simulink model "Commande_7_ReglageCascade_Hinf"  (R2015a)
settings: Solver=ode45  StartTime=0.0  StopTime=20  RelTol=1e-3
values from neighbouring files (symbols this model uses):
  K = place(Aze,Bze,P)    [A_2_Changement_de_base_Diphiomorphisme.m]    (also in A_3_LoopShaping.m = 5000)
  Kd = p1^2*J4    (= 0.0333)    [A_1_Data.m]    (also in matlab.mat = 0.009)
  Kp = -2*p1*J4    (= 0.00222)    [A_1_Data.m]    (also in matlab.mat = 0.0006)
  s = tf('s')    [A_3_LoopShaping.m]    (also in A_4_Hinfini.m = zpk('s'))
  X = [0;0;0;0;0;0;0;0]    [A_1_Data.m]
  Y = [0;0;0;0;0;0;0;0]    [A_1_Data.m]
undefined symbols (not defined in the file or in its folder): Z
libraries: sm_lib x332, nesl_utility x15, simulink x1
(part 8 of 10)

== system Commande_7_ReglageCascade_Hinf/RDelta_SM/RD_SM2/BrasParalelle1/BarreParalleles_2_RIGID/Pice4_Tube_1_RIGID ==
  ReferenceFrame : sm_lib/Frames and Transforms/Reference Frame  BlockFunction=simmechanics.library.frames_transforms.reference_frame
  Solid : sm_lib/Body Elements/Solid  InertiaType=Custom  Mass=0.0056953775725032503  MassUnits=kg  CenterOfMass=[-4.1460122344799134e-11 2.6332345173922464e-08 157.00037492761294]  CenterOfMassUnits=mm  MomentsOfInertia=[46.656669534748204 46.656784060773653 0.060513437161415502]  MomentsOfInertiaUnits=kg*mm^2  ProductsOfInertia=[4.4271388779002391e-06 -1.0344554341986986e-06 -6.5578304138838094e-07]  ProductsOfInertiaUnits=kg*mm^2  DensityBased=on  Density=1000  DensityUnits=kg/(m^3)  GraphicType=FromGeometry  MarkerShape=Sphere  MarkerSize=10  MarkerSizeUnits=m  GraphicVisPropType=SimpleVisualProperties  GraphicDiffuseColor=[0.0 0.0 0.0]  GraphicSpecularColor=[0.5 0.5 0.5 1.0]  GraphicAmbientColor=[0.15 0.15 0.15 1.0]  GraphicEmissiveColor=[1.0 0.0 0.0 1.0]  GraphicShininess=75  GraphicOpacity=1  GeometryShape=FromFile  RectangleSize=[1 1]  RectangleSizeUnits=m  BrickDimensions=[1 1 1]  BrickDimensionUnits=m  CylinderRadius=1  CylinderRadiusUnits=m  CylinderLength=1  CylinderLengthUnits=m  SphereRadius=1  SphereRadiusUnits=m  EllipsoidRadii=[1 1 1]  EllipsoidRadiiUnits=m  ExtrusionCrossSection=[1 1; -1 1; -1 -1; 1 -1]  ExtrusionCrossSectionUnits=m  ExtrusionLength=1  ExtrusionLengthUnits=m  PolygonNumSides=3  PolygonOuterRadius=1  PolygonOuterRadiusUnits=m  ExtGeomFileType=STL  ExtGeomFileName=Pièce4_Tube_Défaut_sldprt.STL  ExtGeomFileUnits=mm  RevolutionCrossSection=[1 1; 1 -1; 2 -1; 2 1]  RevolutionCrossSectionUnits=m  RevolutionExtent=Full  RevolutionAngle=180  RevolutionAngleUnits=deg  BlockFunction=simmechanics.library.body_elements.solid
  F : PMIOPort  Port=1  Side=Left
  connections:
  Solid/RConn1 -- ReferenceFrame/RConn1 -- F/RConn1

== system Commande_7_ReglageCascade_Hinf/RDelta_SM/RD_SM2/BrasParalelle2/BarreParalleles_1_RIGID/Pice4_Extremetees_1_RIGID ==
  ReferenceFrame : sm_lib/Frames and Transforms/Reference Frame  BlockFunction=simmechanics.library.frames_transforms.reference_frame
  Solid : sm_lib/Body Elements/Solid  InertiaType=Custom  Mass=0.0043409919402835973  MassUnits=kg  CenterOfMass=[-6.6394731011390018e-06 -1.3723999560385911 4.9969803448403587]  CenterOfMassUnits=mm  MomentsOfInertia=[0.22208105944838133 0.24049053699814107 0.066049415613599144]  MomentsOfInertiaUnits=kg*mm^2  ProductsOfInertia=[-0.022728057317176146 1.1398156711642886e-07 7.9844492116922665e-07]  ProductsOfInertiaUnits=kg*mm^2  DensityBased=on  Density=1000  DensityUnits=kg/(m^3)  GraphicType=FromGeometry  MarkerShape=Sphere  MarkerSize=10  MarkerSizeUnits=m  GraphicVisPropType=SimpleVisualProperties  GraphicDiffuseColor=[0.59999999999999998 0.59999999999999998 0.59999999999999998]  GraphicSpecularColor=[0.5 0.5 0.5 1.0]  GraphicAmbientColor=[0.15 0.15 0.15 1.0]  GraphicEmissiveColor=[0.0 0.0 0.0 1.0]  GraphicShininess=75  GraphicOpacity=1  GeometryShape=FromFile  RectangleSize=[1 1]  RectangleSizeUnits=m  BrickDimensions=[1 1 1]  BrickDimensionUnits=m  CylinderRadius=1  CylinderRadiusUnits=m  CylinderLength=1  CylinderLengthUnits=m  SphereRadius=1  SphereRadiusUnits=m  EllipsoidRadii=[1 1 1]  EllipsoidRadiiUnits=m  ExtrusionCrossSection=[1 1; -1 1; -1 -1; 1 -1]  ExtrusionCrossSectionUnits=m  ExtrusionLength=1  ExtrusionLengthUnits=m  PolygonNumSides=3  PolygonOuterRadius=1  PolygonOuterRadiusUnits=m  ExtGeomFileType=STL  ExtGeomFileName=Pièce4_Extremetees_Défaut_sldprt.STL  ExtGeomFileUnits=mm  RevolutionCrossSection=[1 1; 1 -1; 2 -1; 2 1]  RevolutionCrossSectionUnits=m  RevolutionExtent=Full  RevolutionAngle=180  RevolutionAngleUnits=deg  BlockFunction=simmechanics.library.body_elements.solid
  F : PMIOPort  Port=1  Side=Left
  connections:
  F/RConn1 -- ReferenceFrame/RConn1 -- Solid/RConn1

== system Commande_7_ReglageCascade_Hinf/RDelta_SM/RD_SM2/BrasParalelle2/BarreParalleles_1_RIGID/Pice4_Extremetees_2_RIGID ==
  ReferenceFrame : sm_lib/Frames and Transforms/Reference Frame  BlockFunction=simmechanics.library.frames_transforms.reference_frame
  Solid : sm_lib/Body Elements/Solid  InertiaType=Custom  Mass=0.0043409919402835973  MassUnits=kg  CenterOfMass=[-6.6394731011390018e-06 -1.3723999560385911 4.9969803448403587]  CenterOfMassUnits=mm  MomentsOfInertia=[0.22208105944838133 0.24049053699814107 0.066049415613599144]  MomentsOfInertiaUnits=kg*mm^2  ProductsOfInertia=[-0.022728057317176146 1.1398156711642886e-07 7.9844492116922665e-07]  ProductsOfInertiaUnits=kg*mm^2  DensityBased=on  Density=1000  DensityUnits=kg/(m^3)  GraphicType=FromGeometry  MarkerShape=Sphere  MarkerSize=10  MarkerSizeUnits=m  GraphicVisPropType=SimpleVisualProperties  GraphicDiffuseColor=[0.59999999999999998 0.59999999999999998 0.59999999999999998]  GraphicSpecularColor=[0.5 0.5 0.5 1.0]  GraphicAmbientColor=[0.15 0.15 0.15 1.0]  GraphicEmissiveColor=[0.0 0.0 0.0 1.0]  GraphicShininess=75  GraphicOpacity=1  GeometryShape=FromFile  RectangleSize=[1 1]  RectangleSizeUnits=m  BrickDimensions=[1 1 1]  BrickDimensionUnits=m  CylinderRadius=1  CylinderRadiusUnits=m  CylinderLength=1  CylinderLengthUnits=m  SphereRadius=1  SphereRadiusUnits=m  EllipsoidRadii=[1 1 1]  EllipsoidRadiiUnits=m  ExtrusionCrossSection=[1 1; -1 1; -1 -1; 1 -1]  ExtrusionCrossSectionUnits=m  ExtrusionLength=1  ExtrusionLengthUnits=m  PolygonNumSides=3  PolygonOuterRadius=1  PolygonOuterRadiusUnits=m  ExtGeomFileType=STL  ExtGeomFileName=Pièce4_Extremetees_Défaut_sldprt.STL  ExtGeomFileUnits=mm  RevolutionCrossSection=[1 1; 1 -1; 2 -1; 2 1]  RevolutionCrossSectionUnits=m  RevolutionExtent=Full  RevolutionAngle=180  RevolutionAngleUnits=deg  BlockFunction=simmechanics.library.body_elements.solid
  F : PMIOPort  Port=1  Side=Left
  connections:
  F/RConn1 -- ReferenceFrame/RConn1 -- Solid/RConn1

== system Commande_7_ReglageCascade_Hinf/RDelta_SM/RD_SM2/BrasParalelle2/BarreParalleles_1_RIGID/Pice4_Tube_1_RIGID ==
  ReferenceFrame : sm_lib/Frames and Transforms/Reference Frame  BlockFunction=simmechanics.library.frames_transforms.reference_frame
  Solid : sm_lib/Body Elements/Solid  InertiaType=Custom  Mass=0.0056953775725032503  MassUnits=kg  CenterOfMass=[-4.1460122344799134e-11 2.6332345173922464e-08 157.00037492761294]  CenterOfMassUnits=mm  MomentsOfInertia=[46.656669534748204 46.656784060773653 0.060513437161415502]  MomentsOfInertiaUnits=kg*mm^2  ProductsOfInertia=[4.4271388779002391e-06 -1.0344554341986986e-06 -6.5578304138838094e-07]  ProductsOfInertiaUnits=kg*mm^2  DensityBased=on  Density=1000  DensityUnits=kg/(m^3)  GraphicType=FromGeometry  MarkerShape=Sphere  MarkerSize=10  MarkerSizeUnits=m  GraphicVisPropType=SimpleVisualProperties  GraphicDiffuseColor=[0.0 0.0 0.0]  GraphicSpecularColor=[0.5 0.5 0.5 1.0]  GraphicAmbientColor=[0.15 0.15 0.15 1.0]  GraphicEmissiveColor=[1.0 0.0 0.0 1.0]  GraphicShininess=75  GraphicOpacity=1  GeometryShape=FromFile  RectangleSize=[1 1]  RectangleSizeUnits=m  BrickDimensions=[1 1 1]  BrickDimensionUnits=m  CylinderRadius=1  CylinderRadiusUnits=m  CylinderLength=1  CylinderLengthUnits=m  SphereRadius=1  SphereRadiusUnits=m  EllipsoidRadii=[1 1 1]  EllipsoidRadiiUnits=m  ExtrusionCrossSection=[1 1; -1 1; -1 -1; 1 -1]  ExtrusionCrossSectionUnits=m  ExtrusionLength=1  ExtrusionLengthUnits=m  PolygonNumSides=3  PolygonOuterRadius=1  PolygonOuterRadiusUnits=m  ExtGeomFileType=STL  ExtGeomFileName=Pièce4_Tube_Défaut_sldprt.STL  ExtGeomFileUnits=mm  RevolutionCrossSection=[1 1; 1 -1; 2 -1; 2 1]  RevolutionCrossSectionUnits=m  RevolutionExtent=Full  RevolutionAngle=180  RevolutionAngleUnits=deg  BlockFunction=simmechanics.library.body_elements.solid
  F : PMIOPort  Port=1  Side=Left
  connections:
  F/RConn1 -- Solid/RConn1 -- ReferenceFrame/RConn1

== system Commande_7_ReglageCascade_Hinf/RDelta_SM/RD_SM2/BrasParalelle2/BarreParalleles_2_RIGID/Pice4_Extremetees_1_RIGID ==
  ReferenceFrame : sm_lib/Frames and Transforms/Reference Frame  BlockFunction=simmechanics.library.frames_transforms.reference_frame
  Solid : sm_lib/Body Elements/Solid  InertiaType=Custom  Mass=0.0043409919402835973  MassUnits=kg  CenterOfMass=[-6.6394731011390018e-06 -1.3723999560385911 4.9969803448403587]  CenterOfMassUnits=mm  MomentsOfInertia=[0.22208105944838133 0.24049053699814107 0.066049415613599144]  MomentsOfInertiaUnits=kg*mm^2  ProductsOfInertia=[-0.022728057317176146 1.1398156711642886e-07 7.9844492116922665e-07]  ProductsOfInertiaUnits=kg*mm^2  DensityBased=on  Density=1000  DensityUnits=kg/(m^3)  GraphicType=FromGeometry  MarkerShape=Sphere  MarkerSize=10  MarkerSizeUnits=m  GraphicVisPropType=SimpleVisualProperties  GraphicDiffuseColor=[0.59999999999999998 0.59999999999999998 0.59999999999999998]  GraphicSpecularColor=[0.5 0.5 0.5 1.0]  GraphicAmbientColor=[0.15 0.15 0.15 1.0]  GraphicEmissiveColor=[0.0 0.0 0.0 1.0]  GraphicShininess=75  GraphicOpacity=1  GeometryShape=FromFile  RectangleSize=[1 1]  RectangleSizeUnits=m  BrickDimensions=[1 1 1]  BrickDimensionUnits=m  CylinderRadius=1  CylinderRadiusUnits=m  CylinderLength=1  CylinderLengthUnits=m  SphereRadius=1  SphereRadiusUnits=m  EllipsoidRadii=[1 1 1]  EllipsoidRadiiUnits=m  ExtrusionCrossSection=[1 1; -1 1; -1 -1; 1 -1]  ExtrusionCrossSectionUnits=m  ExtrusionLength=1  ExtrusionLengthUnits=m  PolygonNumSides=3  PolygonOuterRadius=1  PolygonOuterRadiusUnits=m  ExtGeomFileType=STL  ExtGeomFileName=Pièce4_Extremetees_Défaut_sldprt.STL  ExtGeomFileUnits=mm  RevolutionCrossSection=[1 1; 1 -1; 2 -1; 2 1]  RevolutionCrossSectionUnits=m  RevolutionExtent=Full  RevolutionAngle=180  RevolutionAngleUnits=deg  BlockFunction=simmechanics.library.body_elements.solid
  F : PMIOPort  Port=1  Side=Left
  connections:
  F/RConn1 -- ReferenceFrame/RConn1 -- Solid/RConn1

== system Commande_7_ReglageCascade_Hinf/RDelta_SM/RD_SM2/BrasParalelle2/BarreParalleles_2_RIGID/Pice4_Extremetees_2_RIGID ==
  ReferenceFrame : sm_lib/Frames and Transforms/Reference Frame  BlockFunction=simmechanics.library.frames_transforms.reference_frame
  Solid : sm_lib/Body Elements/Solid  InertiaType=Custom  Mass=0.0043409919402835973  MassUnits=kg  CenterOfMass=[-6.6394731011390018e-06 -1.3723999560385911 4.9969803448403587]  CenterOfMassUnits=mm  MomentsOfInertia=[0.22208105944838133 0.24049053699814107 0.066049415613599144]  MomentsOfInertiaUnits=kg*mm^2  ProductsOfInertia=[-0.022728057317176146 1.1398156711642886e-07 7.9844492116922665e-07]  ProductsOfInertiaUnits=kg*mm^2  DensityBased=on  Density=1000  DensityUnits=kg/(m^3)  GraphicType=FromGeometry  MarkerShape=Sphere  MarkerSize=10  MarkerSizeUnits=m  GraphicVisPropType=SimpleVisualProperties  GraphicDiffuseColor=[0.59999999999999998 0.59999999999999998 0.59999999999999998]  GraphicSpecularColor=[0.5 0.5 0.5 1.0]  GraphicAmbientColor=[0.15 0.15 0.15 1.0]  GraphicEmissiveColor=[0.0 0.0 0.0 1.0]  GraphicShininess=75  GraphicOpacity=1  GeometryShape=FromFile  RectangleSize=[1 1]  RectangleSizeUnits=m  BrickDimensions=[1 1 1]  BrickDimensionUnits=m  CylinderRadius=1  CylinderRadiusUnits=m  CylinderLength=1  CylinderLengthUnits=m  SphereRadius=1  SphereRadiusUnits=m  EllipsoidRadii=[1 1 1]  EllipsoidRadiiUnits=m  ExtrusionCrossSection=[1 1; -1 1; -1 -1; 1 -1]  ExtrusionCrossSectionUnits=m  ExtrusionLength=1  ExtrusionLengthUnits=m  PolygonNumSides=3  PolygonOuterRadius=1  PolygonOuterRadiusUnits=m  ExtGeomFileType=STL  ExtGeomFileName=Pièce4_Extremetees_Défaut_sldprt.STL  ExtGeomFileUnits=mm  RevolutionCrossSection=[1 1; 1 -1; 2 -1; 2 1]  RevolutionCrossSectionUnits=m  RevolutionExtent=Full  RevolutionAngle=180  RevolutionAngleUnits=deg  BlockFunction=simmechanics.library.body_elements.solid
  F : PMIOPort  Port=1  Side=Left
  connections:
  F/RConn1 -- ReferenceFrame/RConn1 -- Solid/RConn1

== system Commande_7_ReglageCascade_Hinf/RDelta_SM/RD_SM2/BrasParalelle2/BarreParalleles_2_RIGID/Pice4_Tube_1_RIGID ==
  ReferenceFrame : sm_lib/Frames and Transforms/Reference Frame  BlockFunction=simmechanics.library.frames_transforms.reference_frame
  Solid : sm_lib/Body Elements/Solid  InertiaType=Custom  Mass=0.0056953775725032503  MassUnits=kg  CenterOfMass=[-4.1460122344799134e-11 2.6332345173922464e-08 157.00037492761294]  CenterOfMassUnits=mm  MomentsOfInertia=[46.656669534748204 46.656784060773653 0.060513437161415502]  MomentsOfInertiaUnits=kg*mm^2  ProductsOfInertia=[4.4271388779002391e-06 -1.0344554341986986e-06 -6.5578304138838094e-07]  ProductsOfInertiaUnits=kg*mm^2  DensityBased=on  Density=1000  DensityUnits=kg/(m^3)  GraphicType=FromGeometry  MarkerShape=Sphere  MarkerSize=10  MarkerSizeUnits=m  GraphicVisPropType=SimpleVisualProperties  GraphicDiffuseColor=[0.0 0.0 0.0]  GraphicSpecularColor=[0.5 0.5 0.5 1.0]  GraphicAmbientColor=[0.15 0.15 0.15 1.0]  GraphicEmissiveColor=[1.0 0.0 0.0 1.0]  GraphicShininess=75  GraphicOpacity=1  GeometryShape=FromFile  RectangleSize=[1 1]  RectangleSizeUnits=m  BrickDimensions=[1 1 1]  BrickDimensionUnits=m  CylinderRadius=1  CylinderRadiusUnits=m  CylinderLength=1  CylinderLengthUnits=m  SphereRadius=1  SphereRadiusUnits=m  EllipsoidRadii=[1 1 1]  EllipsoidRadiiUnits=m  ExtrusionCrossSection=[1 1; -1 1; -1 -1; 1 -1]  ExtrusionCrossSectionUnits=m  ExtrusionLength=1  ExtrusionLengthUnits=m  PolygonNumSides=3  PolygonOuterRadius=1  PolygonOuterRadiusUnits=m  ExtGeomFileType=STL  ExtGeomFileName=Pièce4_Tube_Défaut_sldprt.STL  ExtGeomFileUnits=mm  RevolutionCrossSection=[1 1; 1 -1; 2 -1; 2 1]  RevolutionCrossSectionUnits=m  RevolutionExtent=Full  RevolutionAngle=180  RevolutionAngleUnits=deg  BlockFunction=simmechanics.library.body_elements.solid
  F : PMIOPort  Port=1  Side=Left
  connections:
  F/RConn1 -- Solid/RConn1 -- ReferenceFrame/RConn1

== system Commande_7_ReglageCascade_Hinf/RDelta_SM/RD_SM2/BrasParalelle3/BarreParalleles_1_RIGID/Pice4_Extremetees_1_RIGID ==
  ReferenceFrame : sm_lib/Frames and Transforms/Reference Frame  BlockFunction=simmechanics.library.frames_transforms.reference_frame
  Solid : sm_lib/Body Elements/Solid  InertiaType=Custom  Mass=0.0043409919402835973  MassUnits=kg  CenterOfMass=[-6.6394731011390018e-06 -1.3723999560385911 4.9969803448403587]  CenterOfMassUnits=mm  MomentsOfInertia=[0.22208105944838133 0.24049053699814107 0.066049415613599144]  MomentsOfInertiaUnits=kg*mm^2  ProductsOfInertia=[-0.022728057317176146 1.1398156711642886e-07 7.9844492116922665e-07]  ProductsOfInertiaUnits=kg*mm^2  DensityBased=on  Density=1000  DensityUnits=kg/(m^3)  GraphicType=FromGeometry  MarkerShape=Sphere  MarkerSize=10  MarkerSizeUnits=m  GraphicVisPropType=SimpleVisualProperties  GraphicDiffuseColor=[0.59999999999999998 0.59999999999999998 0.59999999999999998]  GraphicSpecularColor=[0.5 0.5 0.5 1.0]  GraphicAmbientColor=[0.15 0.15 0.15 1.0]  GraphicEmissiveColor=[0.0 0.0 0.0 1.0]  GraphicShininess=75  GraphicOpacity=1  GeometryShape=FromFile  RectangleSize=[1 1]  RectangleSizeUnits=m  BrickDimensions=[1 1 1]  BrickDimensionUnits=m  CylinderRadius=1  CylinderRadiusUnits=m  CylinderLength=1  CylinderLengthUnits=m  SphereRadius=1  SphereRadiusUnits=m  EllipsoidRadii=[1 1 1]  EllipsoidRadiiUnits=m  ExtrusionCrossSection=[1 1; -1 1; -1 -1; 1 -1]  ExtrusionCrossSectionUnits=m  ExtrusionLength=1  ExtrusionLengthUnits=m  PolygonNumSides=3  PolygonOuterRadius=1  PolygonOuterRadiusUnits=m  ExtGeomFileType=STL  ExtGeomFileName=Pièce4_Extremetees_Défaut_sldprt.STL  ExtGeomFileUnits=mm  RevolutionCrossSection=[1 1; 1 -1; 2 -1; 2 1]  RevolutionCrossSectionUnits=m  RevolutionExtent=Full  RevolutionAngle=180  RevolutionAngleUnits=deg  BlockFunction=simmechanics.library.body_elements.solid
  F : PMIOPort  Port=1  Side=Left
  connections:
  Solid/RConn1 -- ReferenceFrame/RConn1 -- F/RConn1

== system Commande_7_ReglageCascade_Hinf/RDelta_SM/RD_SM2/BrasParalelle3/BarreParalleles_1_RIGID/Pice4_Extremetees_2_RIGID ==
  ReferenceFrame : sm_lib/Frames and Transforms/Reference Frame  BlockFunction=simmechanics.library.frames_transforms.reference_frame
  Solid : sm_lib/Body Elements/Solid  InertiaType=Custom  Mass=0.0043409919402835973  MassUnits=kg  CenterOfMass=[-6.6394731011390018e-06 -1.3723999560385911 4.9969803448403587]  CenterOfMassUnits=mm  MomentsOfInertia=[0.22208105944838133 0.24049053699814107 0.066049415613599144]  MomentsOfInertiaUnits=kg*mm^2  ProductsOfInertia=[-0.022728057317176146 1.1398156711642886e-07 7.9844492116922665e-07]  ProductsOfInertiaUnits=kg*mm^2  DensityBased=on  Density=1000  DensityUnits=kg/(m^3)  GraphicType=FromGeometry  MarkerShape=Sphere  MarkerSize=10  MarkerSizeUnits=m  GraphicVisPropType=SimpleVisualProperties  GraphicDiffuseColor=[0.59999999999999998 0.59999999999999998 0.59999999999999998]  GraphicSpecularColor=[0.5 0.5 0.5 1.0]  GraphicAmbientColor=[0.15 0.15 0.15 1.0]  GraphicEmissiveColor=[0.0 0.0 0.0 1.0]  GraphicShininess=75  GraphicOpacity=1  GeometryShape=FromFile  RectangleSize=[1 1]  RectangleSizeUnits=m  BrickDimensions=[1 1 1]  BrickDimensionUnits=m  CylinderRadius=1  CylinderRadiusUnits=m  CylinderLength=1  CylinderLengthUnits=m  SphereRadius=1  SphereRadiusUnits=m  EllipsoidRadii=[1 1 1]  EllipsoidRadiiUnits=m  ExtrusionCrossSection=[1 1; -1 1; -1 -1; 1 -1]  ExtrusionCrossSectionUnits=m  ExtrusionLength=1  ExtrusionLengthUnits=m  PolygonNumSides=3  PolygonOuterRadius=1  PolygonOuterRadiusUnits=m  ExtGeomFileType=STL  ExtGeomFileName=Pièce4_Extremetees_Défaut_sldprt.STL  ExtGeomFileUnits=mm  RevolutionCrossSection=[1 1; 1 -1; 2 -1; 2 1]  RevolutionCrossSectionUnits=m  RevolutionExtent=Full  RevolutionAngle=180  RevolutionAngleUnits=deg  BlockFunction=simmechanics.library.body_elements.solid
  F : PMIOPort  Port=1  Side=Left
  connections:
  Solid/RConn1 -- ReferenceFrame/RConn1 -- F/RConn1

== system Commande_7_ReglageCascade_Hinf/RDelta_SM/RD_SM2/BrasParalelle3/BarreParalleles_1_RIGID/Pice4_Tube_1_RIGID ==
  ReferenceFrame : sm_lib/Frames and Transforms/Reference Frame  BlockFunction=simmechanics.library.frames_transforms.reference_frame
  Solid : sm_lib/Body Elements/Solid  InertiaType=Custom  Mass=0.0056953775725032503  MassUnits=kg  CenterOfMass=[-4.1460122344799134e-11 2.6332345173922464e-08 157.00037492761294]  CenterOfMassUnits=mm  MomentsOfInertia=[46.656669534748204 46.656784060773653 0.060513437161415502]  MomentsOfInertiaUnits=kg*mm^2  ProductsOfInertia=[4.4271388779002391e-06 -1.0344554341986986e-06 -6.5578304138838094e-07]  ProductsOfInertiaUnits=kg*mm^2  DensityBased=on  Density=1000  DensityUnits=kg/(m^3)  GraphicType=FromGeometry  MarkerShape=Sphere  MarkerSize=10  MarkerSizeUnits=m  GraphicVisPropType=SimpleVisualProperties  GraphicDiffuseColor=[0.0 0.0 0.0]  GraphicSpecularColor=[0.5 0.5 0.5 1.0]  GraphicAmbientColor=[0.15 0.15 0.15 1.0]  GraphicEmissiveColor=[1.0 0.0 0.0 1.0]  GraphicShininess=75  GraphicOpacity=1  GeometryShape=FromFile  RectangleSize=[1 1]  RectangleSizeUnits=m  BrickDimensions=[1 1 1]  BrickDimensionUnits=m  CylinderRadius=1  CylinderRadiusUnits=m  CylinderLength=1  CylinderLengthUnits=m  SphereRadius=1  SphereRadiusUnits=m  EllipsoidRadii=[1 1 1]  EllipsoidRadiiUnits=m  ExtrusionCrossSection=[1 1; -1 1; -1 -1; 1 -1]  ExtrusionCrossSectionUnits=m  ExtrusionLength=1  ExtrusionLengthUnits=m  PolygonNumSides=3  PolygonOuterRadius=1  PolygonOuterRadiusUnits=m  ExtGeomFileType=STL  ExtGeomFileName=Pièce4_Tube_Défaut_sldprt.STL  ExtGeomFileUnits=mm  RevolutionCrossSection=[1 1; 1 -1; 2 -1; 2 1]  RevolutionCrossSectionUnits=m  RevolutionExtent=Full  RevolutionAngle=180  RevolutionAngleUnits=deg  BlockFunction=simmechanics.library.body_elements.solid
  F : PMIOPort  Port=1  Side=Left
  connections:
  ReferenceFrame/RConn1 -- Solid/RConn1 -- F/RConn1

== system Commande_7_ReglageCascade_Hinf/RDelta_SM/RD_SM2/BrasParalelle3/BarreParalleles_2_RIGID/Pice4_Extremetees_1_RIGID ==
  ReferenceFrame : sm_lib/Frames and Transforms/Reference Frame  BlockFunction=simmechanics.library.frames_transforms.reference_frame
  Solid : sm_lib/Body Elements/Solid  InertiaType=Custom  Mass=0.0043409919402835973  MassUnits=kg  CenterOfMass=[-6.6394731011390018e-06 -1.3723999560385911 4.9969803448403587]  CenterOfMassUnits=mm  MomentsOfInertia=[0.22208105944838133 0.24049053699814107 0.066049415613599144]  MomentsOfInertiaUnits=kg*mm^2  ProductsOfInertia=[-0.022728057317176146 1.1398156711642886e-07 7.9844492116922665e-07]  ProductsOfInertiaUnits=kg*mm^2  DensityBased=on  Density=1000  DensityUnits=kg/(m^3)  GraphicType=FromGeometry  MarkerShape=Sphere  MarkerSize=10  MarkerSizeUnits=m  GraphicVisPropType=SimpleVisualProperties  GraphicDiffuseColor=[0.59999999999999998 0.59999999999999998 0.59999999999999998]  GraphicSpecularColor=[0.5 0.5 0.5 1.0]  GraphicAmbientColor=[0.15 0.15 0.15 1.0]  GraphicEmissiveColor=[0.0 0.0 0.0 1.0]  GraphicShininess=75  GraphicOpacity=1  GeometryShape=FromFile  RectangleSize=[1 1]  RectangleSizeUnits=m  BrickDimensions=[1 1 1]  BrickDimensionUnits=m  CylinderRadius=1  CylinderRadiusUnits=m  CylinderLength=1  CylinderLengthUnits=m  SphereRadius=1  SphereRadiusUnits=m  EllipsoidRadii=[1 1 1]  EllipsoidRadiiUnits=m  ExtrusionCrossSection=[1 1; -1 1; -1 -1; 1 -1]  ExtrusionCrossSectionUnits=m  ExtrusionLength=1  ExtrusionLengthUnits=m  PolygonNumSides=3  PolygonOuterRadius=1  PolygonOuterRadiusUnits=m  ExtGeomFileType=STL  ExtGeomFileName=Pièce4_Extremetees_Défaut_sldprt.STL  ExtGeomFileUnits=mm  RevolutionCrossSection=[1 1; 1 -1; 2 -1; 2 1]  RevolutionCrossSectionUnits=m  RevolutionExtent=Full  RevolutionAngle=180  RevolutionAngleUnits=deg  BlockFunction=simmechanics.library.body_elements.solid
  F : PMIOPort  Port=1  Side=Left
  connections:
  Solid/RConn1 -- ReferenceFrame/RConn1 -- F/RConn1

== system Commande_7_ReglageCascade_Hinf/RDelta_SM/RD_SM2/BrasParalelle3/BarreParalleles_2_RIGID/Pice4_Extremetees_2_RIGID ==
  ReferenceFrame : sm_lib/Frames and Transforms/Reference Frame  BlockFunction=simmechanics.library.frames_transforms.reference_frame
  Solid : sm_lib/Body Elements/Solid  InertiaType=Custom  Mass=0.0043409919402835973  MassUnits=kg  CenterOfMass=[-6.6394731011390018e-06 -1.3723999560385911 4.9969803448403587]  CenterOfMassUnits=mm  MomentsOfInertia=[0.22208105944838133 0.24049053699814107 0.066049415613599144]  MomentsOfInertiaUnits=kg*mm^2  ProductsOfInertia=[-0.022728057317176146 1.1398156711642886e-07 7.9844492116922665e-07]  ProductsOfInertiaUnits=kg*mm^2  DensityBased=on  Density=1000  DensityUnits=kg/(m^3)  GraphicType=FromGeometry  MarkerShape=Sphere  MarkerSize=10  MarkerSizeUnits=m  GraphicVisPropType=SimpleVisualProperties  GraphicDiffuseColor=[0.59999999999999998 0.59999999999999998 0.59999999999999998]  GraphicSpecularColor=[0.5 0.5 0.5 1.0]  GraphicAmbientColor=[0.15 0.15 0.15 1.0]  GraphicEmissiveColor=[0.0 0.0 0.0 1.0]  GraphicShininess=75  GraphicOpacity=1  GeometryShape=FromFile  RectangleSize=[1 1]  RectangleSizeUnits=m  BrickDimensions=[1 1 1]  BrickDimensionUnits=m  CylinderRadius=1  CylinderRadiusUnits=m  CylinderLength=1  CylinderLengthUnits=m  SphereRadius=1  SphereRadiusUnits=m  EllipsoidRadii=[1 1 1]  EllipsoidRadiiUnits=m  ExtrusionCrossSection=[1 1; -1 1; -1 -1; 1 -1]  ExtrusionCrossSectionUnits=m  ExtrusionLength=1  ExtrusionLengthUnits=m  PolygonNumSides=3  PolygonOuterRadius=1  PolygonOuterRadiusUnits=m  ExtGeomFileType=STL  ExtGeomFileName=Pièce4_Extremetees_Défaut_sldprt.STL  ExtGeomFileUnits=mm  RevolutionCrossSection=[1 1; 1 -1; 2 -1; 2 1]  RevolutionCrossSectionUnits=m  RevolutionExtent=Full  RevolutionAngle=180  RevolutionAngleUnits=deg  BlockFunction=simmechanics.library.body_elements.solid
  F : PMIOPort  Port=1  Side=Left
  connections:
  Solid/RConn1 -- ReferenceFrame/RConn1 -- F/RConn1

== system Commande_7_ReglageCascade_Hinf/RDelta_SM/RD_SM2/BrasParalelle3/BarreParalleles_2_RIGID/Pice4_Tube_1_RIGID ==
  ReferenceFrame : sm_lib/Frames and Transforms/Reference Frame  BlockFunction=simmechanics.library.frames_transforms.reference_frame
  Solid : sm_lib/Body Elements/Solid  InertiaType=Custom  Mass=0.0056953775725032503  MassUnits=kg  CenterOfMass=[-4.1460122344799134e-11 2.6332345173922464e-08 157.00037492761294]  CenterOfMassUnits=mm  MomentsOfInertia=[46.656669534748204 46.656784060773653 0.060513437161415502]  MomentsOfInertiaUnits=kg*mm^2  ProductsOfInertia=[4.4271388779002391e-06 -1.0344554341986986e-06 -6.5578304138838094e-07]  ProductsOfInertiaUnits=kg*mm^2  DensityBased=on  Density=1000  DensityUnits=kg/(m^3)  GraphicType=FromGeometry  MarkerShape=Sphere  MarkerSize=10  MarkerSizeUnits=m  GraphicVisPropType=SimpleVisualProperties  GraphicDiffuseColor=[0.0 0.0 0.0]  GraphicSpecularColor=[0.5 0.5 0.5 1.0]  GraphicAmbientColor=[0.15 0.15 0.15 1.0]  GraphicEmissiveColor=[1.0 0.0 0.0 1.0]  GraphicShininess=75  GraphicOpacity=1  GeometryShape=FromFile  RectangleSize=[1 1]  RectangleSizeUnits=m  BrickDimensions=[1 1 1]  BrickDimensionUnits=m  CylinderRadius=1  CylinderRadiusUnits=m  CylinderLength=1  CylinderLengthUnits=m  SphereRadius=1  SphereRadiusUnits=m  EllipsoidRadii=[1 1 1]  EllipsoidRadiiUnits=m  ExtrusionCrossSection=[1 1; -1 1; -1 -1; 1 -1]  ExtrusionCrossSectionUnits=m  ExtrusionLength=1  ExtrusionLengthUnits=m  PolygonNumSides=3  PolygonOuterRadius=1  PolygonOuterRadiusUnits=m  ExtGeomFileType=STL  ExtGeomFileName=Pièce4_Tube_Défaut_sldprt.STL  ExtGeomFileUnits=mm  RevolutionCrossSection=[1 1; 1 -1; 2 -1; 2 1]  RevolutionCrossSectionUnits=m  RevolutionExtent=Full  RevolutionAngle=180  RevolutionAngleUnits=deg  BlockFunction=simmechanics.library.body_elements.solid
  F : PMIOPort  Port=1  Side=Left
  connections:
  ReferenceFrame/RConn1 -- Solid/RConn1 -- F/RConn1

== matlab function Commande_7_ReglageCascade_Hinf/RDelta_SM/4me_degree/equations electriques ==
  data: I input; U input; dI output; dTheta input
function dI = fcn(I,U,dTheta)

b1 = -1.1250e+03 ;
b2 = -99.4718 ;
b3 =833.3333 ;

dI = b2*dTheta + b1*I + b3*U ;

== matlab function Commande_7_ReglageCascade_Hinf/Trajctoir2/Trajectoir1 ==
  data: Segma output; ne input; P output; dP output; d2P output; t input; d3P output
function [Segma, P,dP,d2P,d3P]= fcn(ne,t)

%% Menu
% 1 ==> Ligne horizontal
% 2==>  Ligne suivant l'axe oz
% 3==> Cercle
% 4==> Ligne x=y
z0= -0.2 ; zpi=-0.35;
B= (z0+zpi)/2 ; A= (z0-zpi)/2 ; 
f = 3; f2 = 5 ;
R=0.25;
%% vers le Plan Z=-0.3
if (t<pi/f && (ne == 1 || ne == 3 ||  ne == 0 || ne == 4 || ne == 5 ||  ne == 6)) % vers le plans z = zpi
n= 2 ; 
elseif( (ne == 4 || ne == 5 ||  ne == 6)  &&  (t<3*pi/2/f) ) % vers le point (0 , R , zpi)
n=1 ;
else
n =ne ;
end

%% le trajecoir
switch n
    
    case 0
        
        % La position
        x = R*sin(f*t)  ; y=0 ;
        z=  zpi ;
        P = [ x ; y ; z ];
        % La vitess
        dx = f*R*cos(f*t)  ; dy=0 ;
        dz= 0 ;
        dP = [ dx ; dy ; dz ];
        % L'acceleration :
        d2x = -f^2*R*sin(f*t) ; d2y=0 ;
        d2z =  0;
        d2P = [ d2x ; d2y ; d2z ];
        % L'a _coup :
        d3x = -f^3*R*cos(f*t) ; d3y=0 ;
        d3z =  0;
        d3P = [ d3x ; d3y ; d3z ];
        Segma = 2*pi*sin(f*t/2) ;
    case 1   
        % La position
        y = R*sin(f*t)  ; x=0 ;
        z= zpi  ;
        P = [ x ; y ; z ];
        % La vitess
        dy = f*R*cos(f*t)  ; dx=0 ;
        dz= 0 ;
        dP = [ dx ; dy ; dz ];
        % L'acceleration :
        d2y = -f^2*R*sin(f*t) ; d2x=0 ;
        d2z =  0;
        d2P = [ d2x ; d2y ; d2z ];
        % L'a _coup :
        d3y = -f^3*R*cos(f*t) ; d3x=0 ;
        d3z =  0;
        d3P = [ d3x ; d3y ; d3z ];
        Segma = pi*sin(f*t) + 2*pi ;
    case 2
        % La position 
        x = 0 ; y=0 ;
        z = A*cos(f*t) + B ; 
        P = [ x ; y ; z ];
        % La vitess
        dx = 0 ; dy=0 ;
        dz= -f*A*sin(f*t) ;
        dP = [ dx ; dy ; dz ];
        % L'acceleration :
        d2x = 0 ; d2y=0 ;
        d2z = -f^2*A*cos(f*t) ;
        d2P = [ d2x ; d2y ; d2z ];
        % L a_coup (jerk) :
        d3x = 0 ; d3y=0 ;
        d3z = f^3*A*sin(f*t) ;
        d3P = [ d3x ; d3y ; d3z ];
        Segma = 2*pi*sin(f*t/2) ;
        
        %%
    case 3
        R=0.12;
        y = R*sin(f*t)  ; x=2*y;
        z= zpi  ;
        P = [ x ; y ; z ];
        % La vitess
        dy = f*R*cos(f*t)  ; dx=2*dy ;
        dz= 0 ;
        dP = [ dx ; dy ; dz ];
        % L'acceleration :
        d2y = -f^2*R*sin(f*t) ; d2x=2*d2y ;
        d2z =  0;
        d2P = [ d2x ; d2y ; d2z ];
        % L'a _coup :
        d3y = -f^3*R*cos(f*t) ; d3x=2*d3y ;
        d3z =  0;
        d3P = [ d3x ; d3y ; d3z ];
        Segma = 2*pi*sin(f*t/2) ;
    case 4 % Cerecl XY
        x=R*cos(f*t) ; y=R*sin(f*t) ; z=zpi  ;
        dx=-f*R*sin(f*t) ; dy=f*R*cos(f*t)  ;  dz=0;
        d2x=-f^2*R*cos(f*t) ; d2y=-f^2*R*sin(f*t)  ;  d2z=0;
        P=[x ; y ; z];
        dP=[dx ; dy ; dz];
        d2P=[d2x ; d2y ; d2z];
        % L'a _coup :
        d3x=f^3*R*sin(f*t) ; d3y=-f^3*R*cos(f*t)  ;  d3z=0;
        d3P=[d3x ; d3y ; d3z];
        Segma = pi -(f*t-3*pi/2) ;
    case 5 % ZY   
        x=0 ; y=R*sin(f*t) ; z=0.5*R*cos(f*t) + zpi  ;
        dx=0 ; dy=f*R*cos(f*t)  ;  dz=-f*R*sin(f*t);
        d2x=0 ; d2y=-f^2*R*sin(f*t)  ;  d2z=-f^2*R*cos(f*t);
        P=[x ; y ; z];
        dP=[dx ; dy ; dz];
        d2P=[d2x ; d2y ; d2z];
        d3x=0 ; d3y=-f^3*R*cos(f*t)  ;  d3z=f^3*R*sin(f*t);
        d3P=[d3x ; d3y ; d3z];
        Segma = 2*pi*sin(f*t/2) ;
%     case 6 %Cercle ZX
%         y=0 ; x=R*sin(f*t) ; z=R*cos(f*t) +zpi;
%         dy=0 ; dx=f*R*cos(f*t)  ;  dz=-f*R*sin(f*t);
%         d2y=0 ; d2x=-f^2*R*sin(f*t)  ;  d2z=-f^2*R*cos(f*t);
%         d3y=0 ; d3x=-f^3*R*cos(f*t)  ;  d3z=f^3*R*sin(f*t);
%         P=[x ; y ; z];
%         dP=[dx ; dy ; dz];
%         d2P=[d2x ; d2y ; d2z];
%         d3P = [ d3x ; d3y ; d3z ];
%     case 7  % Les derivees sont a corriger
%         R=0.00*sin(f2*t) ; A=0.1270 ;
%         x=R*cos(f*t) ; y=R*sin(f*t) ;
%         z= A*sin(f2*t) -0.2 ;
%         dx=-f*R*sin(f*t) ; dy=f*R*cos(f*t)  ;  
%         dz= f2*A*cos(f2*t) ;
%         d2x=-f^2*R*cos(f*t) ; d2y=-f^2*R*sin(f*t)  ;
%         d2z = -f2^2*A*sin(f2*t) ;
%         P=[x ; y ; z];
%         dP=[dx ; dy ; dz];
%         d2P=[d2x ; d2y ; d2z];
%         % L'a _coup :
%         d3x=f^3*R*sin(f*t) ; d3y=-f^3*R*cos(f*t)  ;
%         d3z = -f2^3*A*cos(f2*t) ;
%         d3P=[d3x ; d3y ; d3z];
    case 8
        x=0 ; y=0 ; z=z0 ;
        P=[x ; y ; z];
        dP=[0 ; 0 ; 0];
        d2P=[0 ; 0 ; 0];
        d3P=[0 ; 0 ; 0];
        Segma = 2*pi*sin(f*t/2) ;
    otherwise
        P=[0 ; 0 ; 0];
        dP=[0 ; 0 ; 0];
        d2P=[0 ; 0 ; 0];
        d3P = [ 0 ; 0 ; 0 ];
        Segma = 0 ;
end

== matlab function Commande_7_ReglageCascade_Hinf/Regulateur de la partie mecanique -Hinfini-/Decoupleur1 ==
  data: Q input; DT_ output; R input; Z input; V input; DX1 input; DX2 input
function DT_ = fcn(Q,R,Z, V,DX1,DX2)


Qd = diag(diag(Q)) ; Qd_= Q - Qd ;
Rd = diag(diag(R)) ; Rd_= R - Rd ;
DT_ = Z\(V - Qd_*DX1 - Rd_*DX2) ;

== matlab function Commande_7_ReglageCascade_Hinf/RDelta_SM/Moteurs/equations electriques ==
  data: I input; U input; dI output; dTheta input
function dI = fcn(I,U,dTheta)

b1 = -1.1250e+03 ;
b2 = -99.4718 ;
b3 =833.3333 ;

dI = b2*dTheta + b1*I + b3*U ;

== matlab function Commande_7_ReglageCascade_Hinf/Trajctoir2/Trajectoir2 ==
  data: DP input; i input; t0 input; n input; S input; Segma input; DPP output; ii output; tt0 output; nn output; SS output; Segma_ output; P input; P_ output; dP input; d2P input; d3P input; dP_ output; d2P_ output; d3P_ output; t input
function [DPP,ii,tt0,nn,SS,Segma_,P_,dP_,d2P_,d3P_]= fnc(DP,i,t0,n,S,Segma,P,dP,d2P,d3P,t)

%% Constante
f= 3 ;  zpi=-0.35; ee=0.00001 ;
nn=n;
SS=S ;
tt0= t0;
Dt = t-t0 ;
Di=1;
%% les positions des pieces sur le cercle
X = [ 0.2500; 0.1768; 0.0000; -0.1768; -0.2500; -0.1768; -0.0000; 0.1768 ] ;
Y =[ 0; 0.1768; 0.2500;  0.1768; 0.0000; -0.1768; -0.2500; -0.1768] ;
% les angles des pieces
SEGMA=[pi/2 ;pi/4 ; 0 ; -pi/4 ; -pi/2 ; -3*pi/4 ; -pi ; -5*pi/4] ;



%% le depart et l'arrivee du trajectoir (cercle)
x0 = X( 8*not(mod(i,8))+mod(i,8)) ;
y0=Y(8*not(mod(i,8))+mod(i,8));
x1 = X(8*not(mod(i+Di,8))+mod(i+Di,8)) ;
y1=Y(8*not(mod(i+Di,8))+mod(i+Di,8));
%% le depart et l'arrivee du 4 degree (Cercle)
S0=SEGMA(8*not(mod(i,8))+mod(i,8));
S1= SEGMA(8*not(mod(i+Di,8))+mod(i+Di,8)) ;
%% les positions des pieces sur ENP
Xenp = [0.2500   -0.0900    0.1768   -0.1200         0   -0.0900   -0.1768   -0.1200   -0.2500   -0.0900   -0.1768   -0.0300         0   -0.0300    0.1768         0    0.2500    0.0300    0.1768    0.0300    0    0.0700   -0.1768    0.0700   -0.2500    0.1000   -0.1768    0.1300         0    0.1000  ]' ;
Yenp=[0    0.0500    0.1768    0.0250    0.2500         0    0.1768   -0.0250         0   -0.0500 -0.1768   -0.0250   -0.2500    0.0250   -0.1768         0         0   -0.0250    0.1768    0.0250  0.2500   -0.0250    0.1768    0.0250         0    0.0500   -0.1768    0.0250   -0.2500         0 ]';
% les angles des pieces
SEGMAenp=[  1.5708    1.5708    0.7854         0         0    1.5708   -0.7854         0   -1.5708  1.5708   -2.3562         0   -3.1416         0   -3.9270    -0.5400    1.5708         0   0.7854         0         0         0   -0.7854         0   -1.5708    1.5708   -2.3562    0   -3.1416    1.5708]' ; 
x0 = Xenp( 30*not(mod(i,30))+mod(i,30)) ;
y0=Yenp(30*not(mod(i,30))+mod(i,30));
x1 = Xenp(30*not(mod(i+Di,30))+mod(i+Di,30)) ;
y1=Yenp(30*not(mod(i+Di,30))+mod(i+Di,30));
%% le depart et l'arrivee du 4 degree (Cercle)
S0=SEGMAenp(30*not(mod(i,30))+mod(i,30));
S1= SEGMAenp(30*not(mod(i+Di,30))+mod(i+Di,30)) ;

%% les rayons du trajectoir
R = sqrt((x1-x0)^2 + (y1-y0)^2)/2  ;
Rz = 0.5*R ;
%   
ii=i ;
if (t<(3*pi/2/f + 2*pi/f))
P_=P ; dP_=dP ; d2P_=d2P ; d3P_=d3P ; 
Segma_=Segma ;
else
   
     e=R*cos(f*Dt) ; z=Rz*sin(f*Dt) + zpi  ;
     de=-f*R*sin(f*Dt)  ;  dz=f*Rz*cos(f*Dt);
     d2e=-f^2*R*cos(f*Dt)  ;  d2z=-f^2*Rz*sin(f*Dt);
     d3e=f^3*R*sin(f*Dt)  ;  d3z=-f^3*Rz*cos(f*Dt);
     Cn=(x1-x0)/R/2 ; Sn= (y1-y0)/R /2;
     x=x0 + (R-e)*Cn;
     y=y0 + (R-e)*Sn;
     dx=-de*Cn; dy = -de*Sn ;
     d2x=-d2e*Cn ; d2y = -d2e*Sn ;
     d3x=-d3e*Cn; d3y = -d3e*Sn ;
     
        P_=[x ;  y ; z];
        dP_=[dx ; dy ; dz];
        d2P_=[d2x ; d2y ; d2z];
        d3P_=[d3x ; d3y ; d3z];
        DS=S1-S0;
        Segma_ = S + DS*sin(f*Dt/2); 
     
        if (abs(DP(1))<ee && abs(DP(2))<ee && n==1 )
                          
            ii=i+Di ;   tt0 =  t ;
                           nn=0 ; SS=Segma_ ;
                           else if ((abs(DP(1))>ee || abs(DP(2))>ee) && n==0)
                                   nn= 1;
                               end
        end
           
end

DPP = [ P_(1) - x1 ; P_(2) - y1 ] ;



% %% les positions des pieces sur ENP
% Xenp = [ -90;-120 ;-90 ;-120 ;-90 ;-30 ;-30 ;0; 30; 30; 70;70 ;100 ;130;100 ]/1000 ;
% Yenp = [ 50;25 ; 0 ; -25; -50; -25; 25 ; 0 ;-25 ;25 ; -25 ; 25 ; 50 ; 25 ;0 ]/1000 ;
% % les angles des pieces
% SEGMAenp=[pi/2 ; 0  ;pi/2 ; 0 ; pi/2; 0;0  ;-0.54 ;0 ;0 ;0 ;0 ;pi/2 ;0 ;pi/2 ] ;

== matlab function Commande_7_ReglageCascade_Hinf/Point de foncitonnnement/Calcule de Q R Z  ==
  data: dT_Theta input; dT_dTheta input; dT_d2Theta input; Q output; R output; Z output
function [Q,R,Z]= fcn(dT_Theta,dT_dTheta,dT_d2Theta )

Z = eye(3,3)/ dT_d2Theta ;
Q= -Z*dT_Theta ;
R=-Z*dT_dTheta ;
%d3Theta = Q*dTheta + R*d2Theta + Z*dT ;

== matlab function Commande_7_ReglageCascade_Hinf/Point de foncitonnnement/Derivee de Tg/Gravite_lineaire ==
  data: Tg output; P input; alpha input; dTg_Theta output; Jinv input
function [Tg,dTg_Theta]= fcn(P,alpha,Jinv)

    alpha1=alpha(1) ;alpha2=alpha(2) ; alpha3=alpha(3) ;
    
%% les constantes:
l1 = 0.19992; 
l2 = 0.334; 
r = 0.126; 
phi2 = 2*pi/3;
phi3 = 4*pi/3;
A2=[cos(phi2) sin(phi2) 0 
     -sin(phi2) cos(phi2) 0
        0            0            1 ]; 
A3=[cos(phi3) sin(phi3) 0
     -sin(phi3) cos(phi3) 0
          0            0          1 ];
g = 9.98 ;
mBras = 0.083660682814532691 ;
mRoue =0.1805;
dBras = 0.058869490365843639 ;
dRoue = 0.0344586;
M2= 2*0.01438 ;
M3 = 0.0416;
shift = 0.0651;
%% Parametres :
    % A) les vecteurs OAi et OBi :
    OA1=[r ; 0 ; 0] ; OA2=[r*cos(phi2) ; r*sin(phi2) ; 0] ; OA3=[r*cos(phi3) ; r*sin(phi3) ; 0] ;
    OC1=[r+l1*cos(alpha1) ; 0 ; -l1*sin(alpha1) ]; 
    OC2=[(r+l1*cos(alpha2))*cos(phi2) ; (r+l1*cos(alpha2))*sin(phi2) ; -l1*sin(alpha2) ]; 
    OC3=[(r+l1*cos(alpha3))*cos(phi3) ; (r+l1*cos(alpha3))*sin(phi3) ; -l1*sin(alpha3) ]; 
    % B) Les vecteurs AiCi :
    A1C1=OC1-OA1 ; A2C2=OC2-OA2 ; A3C3=OC3-OA3 ;
    % Fin

%% ===============-------=====  Calcule de Cgi =====---------====================

% Les vecteurs unitaires portes par les bras paralleles : la nouvelle base
    u1=(P-OC1)/l2 ; u2=(P-OC2)/l2 ; u3=(P-OC3)/l2 ;
    U = [u1 u2 u3] ;

% Les forces aux points Ci ;
     N1=[-dBras*mBras*sin(shift) - dRoue*mRoue*cos(shift) ; 0 ; -dBras*mBras*cos(shift) + dRoue*mRoue*sin(shift)]*g/l1; 
    N2=[0 ;0 ; -M2*g/2] ;
    N=N1+N2;

% les effets totales appliquees a  la nacelle (N4):
    N4 = [0 ; 0 ; -(M3 + M2*3/2)*g] ;

% les composants de N4 sur les bras paralleles = Expression de N4 dans la Nouvelle base U:
    E1 = [1 0 0]; E2 = [0 1 0]; E3 = [0 0 1];
    Z = U\N4 ;
    Z1=(E1*Z)*u1; 
    Z2=(E2*Z)*u2;  
    Z3=(E3*Z)*u3 ;

% les matrices de transformation au plan OXiZi (Bi) :
    B1= [1 0 0; 0 0 0 ; 0 0 1] ;
    B2=B1*A2; B3=B1*A3 ;
% Le couple Cg1 au point de fonc P0:
Cg1 = E2*cross(A1C1,N + B1*Z1);
Cg2 = E2* cross(A2*A2C2,N + B2*Z2)  ;
Cg3 = E2* cross(A3*A3C3, N + B3*Z3) ;
Cg =[Cg1 ;Cg2;Cg3] ;
Tg=Cg/12 ;
%% =========================== Linearisation ================================

% A) la derivee de ACi par rapport au alphai
    dAC1_1=[-l1*sin(alpha1) ; 0 ; -l1*cos(alpha1) ] ; 
    dAC2_2=A2'*[-l1*sin(alpha2); 0 ; -l1*cos(alpha2) ] ;
    dAC3_3=A3'*[-l1*sin(alpha3); 0 ; -l1*cos(alpha3)] ;

% B) les derivees partielles de la matrice U  par rapport au Apha_i
    % les derivees partielles de u1 par rapport au alphai
    du1_1=(Jinv*E1'-dAC1_1)/l2 ; 
    du1_2=(Jinv*E2')/l2 ; 
    du1_3=(Jinv*E3')/l2 ;
    % les derivees partielles de u2 par rapport au alphai
    du2_1=(Jinv*E1')/l2 ; 
    du2_2=(Jinv*E2'-dAC2_2)/l2 ; 
    du2_3=du1_3 ;
    % la derivee partielle de u3 par rapport au alphai
    du3_1=du2_1; 
    du3_2=du1_2; 
    du3_3=(Jinv*E3'-dAC3_3)/l2 ;
    % finalement
    dU_1=[du1_1 , du2_1 , du3_1]; % la derivee partielle de la matrice U par rapport au alpha1
    dU_2=[du1_2 , du2_2 , du3_2]; % la derivee partielle de la matrice U par rapport au alpha2
    dU_3=[du1_3 , du2_3 , du3_3]; % la derivee partielle de la matrice U par rapport au alpha3
    %dU = dU_1*dalpha(1) + dU_2*dalpha(2) +dU_3*dalpha(3) ;

% C) les derivees partielles de Z par rapport au alpha_i
    dZ_1=-U\dU_1*Z ;
    dZ_2=-U\dU_2*Z ;
    dZ_3=-U\dU_3*Z ;
    %dZ=dZ_1*Dalpha(1)+ dZ_2*Dalpha(2) + dZ_3*Dalpha(3) ;

% D) les derivee partilles de Zi par rapport au alpha_i :
    % La derivee de Z1 par rapport au alphai
    dZ1_1 = (E1*dZ_1)*u1+(E1*Z)*du1_1 ;
    dZ1_2 = (E1*dZ_2)*u1+(E1*Z)*du1_2 ;
    dZ1_3 = (E1*dZ_3)*u1+(E1*Z)*du1_3 ;
    % La derivee de Z2 par rapport au alphai
    dZ2_1 = (E2*dZ_1)*u2+(E2*Z)*du2_1 ;
    dZ2_2 = (E2*dZ_2)*u2+(E2*Z)*du2_2 ;
    dZ2_3 = (E2*dZ_3)*u2+(E2*Z)*du2_3 ;
    % La derivee de Z3 par rapport au alphai
    dZ3_1 = (E3*dZ_1)*u3+(E3*Z)*du3_1 ;
    dZ3_2 = (E3*dZ_2)*u3+(E3*Z)*du3_2 ;
    dZ3_3 = (E3*dZ_3)*u3+(E3*Z)*du3_3 ;
    %dZ3=dZ3_1*dalpha(1)+ dZ3_2*dalpha(2) + dZ3_3*dalpha(3) ;

%% E) les derivees partilles de Cgi par rapport au alpha_i :

    % 1) Les derivees partielles de Cg1:
    dCg1_1 = E2* cross(dAC1_1, N + B1*Z1) + E2*cross(A1C1 , B1*dZ1_1) ;
    dCg1_2 = E2*cross(A1C1 , B1*dZ1_2) ;
    dCg1_3 = E2*cross(A1C1 , B1*dZ1_3) ;
    dCg1_alpha = [dCg1_1 , dCg1_2 , dCg1_3] ; % dimension :1*3
    %dCg1= dCg1_1*Dalpha(1) + dCg1_2*Dalpha(2)  + dCg1_3*Dalpha(3) ;
    
    % 2) Les derivees partielles de Cg2:
    dCg2_1 = E2*cross(A2*A2C2 , B2*dZ2_1) ;
    dCg2_2 = E2* cross(A2*dAC2_2, N + B2*Z2) + E2*cross(A2*A2C2 , B2*dZ2_2) ;
    dCg2_3 = E2*cross(A2*A2C2 , B2*dZ2_3) ;
    dCg2_alpha = [dCg2_1 , dCg2_2 , dCg2_3] ;
    %dCg2= dCg2_1*Dalpha(1) + dCg2_2*Dalpha(2)  +dCg2_3*Dalpha(3) ;

    % 3) Les derivees partielles de Cg3:
    dCg3_1 = E2*cross(A3*A3C3 , B3*dZ3_1) ;
    dCg3_2 = E2*cross(A3*A3C3 , B3*dZ3_2) ;
    dCg3_3 = E2*cross(A3*dAC3_3, N + B3*Z3) + E2*cross(A3*A3C3 , B3*dZ3_3) ;
    dCg3_alpha = [dCg3_1 , dCg3_2 , dCg3_3] ;
    %dCg3= dCg3_1*Dalpha(1) + dCg3_2*Dalpha(2)  +dCg3_3*Dalpha(3) ;

dCg_alpha = [dCg1_alpha;dCg2_alpha;dCg3_alpha] ;

%% Les derivees partielles de Tg :
%Theta = alpha*12 ; dTheta = dalpha*12 ; 
dTg_Theta = dCg_alpha/12^2 ; %% RQ :dTg_Theta = dTg_alpha/12
%dTg = dTg_Theta * dTheta ;

== matlab function Commande_7_ReglageCascade_Hinf/Point de foncitonnnement/Derivee de Tg/Jinv ==
  data: P input; Jinv output
function Jinv= fcn(P)

l1 = 0.19992; 
l2 = 0.334; 
r = 0.126; 
phi2 = 2*pi/3;
phi3 = 4*pi/3;

%% projection de P sur Ri
A2=[cos(phi2) sin(phi2) 0
    -sin(phi2) cos(phi2) 0
    0            0      1 ]; 
A3=[cos(phi3) sin(phi3) 0
    -sin(phi3) cos(phi3) 0
    0            0      1 ];
P2=A2*P; P3=A3*P ;

x1=P(1); y1=P(2) ; z1=P(3) ; %% p1=p
x2=P2(1); y2=P2(2) ; z2=P2(3) ;
x3=P3(1); y3=P3(2) ; z3=P3(3) ;

%% Calcule de ABi et ei :
AB1=sqrt(z1^2+(x1-r)^2);
e1=sqrt(l2^2-y1^2); 
AB2=sqrt(z2^2+(x2-r)^2);
e2=sqrt(l2^2-y2^2);
AB3=sqrt(z3^2+(x3-r)^2);
e3=sqrt(l2^2-y3^2);

%% calcul de alpha1
gama1=acos((AB1^2 + l1^2 - e1^2)/(2*l1*AB1));
gama2=acos((AB2^2 + l1^2 - e2^2)/(2*l1*AB2));
gama3=acos((AB3^2 + l1^2 - e3^2)/(2*l1*AB3));

%% =========== Calcule de  J1  ================
% J1 est defini par : dalpha1= J1*dP
AB1 = sqrt(z1^2+(x1-r)^2);
AH1 = AB1-l1*cos(gama1);
D1=1/(l1*AB1*sin(gama1));
a1 = D1*AH1*(x1-r)/AB1 +  z1/( z1^2 + (x1-r)^2 );
a2 = D1*y1 ;
a3 = D1*AH1*z1/AB1 -(x1-r)/( z1^2 + (x1-r)^2 ) ;
j1= [a1 a2 a3] ;

%% =========== Calcule de  J2  ================
% J2 est defini par : dalpha2 = J2*A2*dP
AB2 = sqrt(z2^2+(x2-r)^2);
AH2 = AB2-l1*cos(gama2);
D2=1/(l1*AB2*sin(gama2));
a4 = D2*AH2*(x2-r)/AB2 + z2/( z2^2 + (x2-r)^2 ) ;
a5 = D2*y2;
a6 = D2*AH2*z2/AB2 -(x2-r)/( z2^2 + (x2-r)^2 );
j2=[a4 a5 a6]*A2;

%%  ========= (dAlpha3)  ================

AB3 = sqrt(z3^2+(x3-r)^2);
AH3 = AB3-l1*cos(gama3);
D3=1/(l1*AB3*sin(gama3));
a7 = D3*AH3*(x3-r)/AB3 + z3/( z3^2 + (x3-r)^2 );
a8 = D3*y3;
a9 = D3*AH3*z3/AB3 -(x3-r)/( z3^2 + (x3-r)^2 ) ;
j3=[ a7 a8 a9]*A3 ;

%% La matrice inverse de J
J=[ j1 ; j2 ; j3 ];
%  dAlpha=J*dp;   
Jinv=eye(3,3) /J;

== matlab function Commande_7_ReglageCascade_Hinf/Point de foncitonnnement/La tension et le Courant au point de fonctionnement ==
  data: U output; T input; dT input; dTheta input; I output
function [U,I]= fcn(T,dT,dTheta)

b1 = -1.1250e+03 ;
b2 = -99.4718 ;
b3 =833.3333 ;
Ki=0.119 ;
I = T/Ki ;
dI = dT/Ki ;
U = (dI - b2*dTheta - b1*I)/b3 ;

== matlab function Commande_7_ReglageCascade_Hinf/RDelta_SM/Regulateur De 4 eme degree/Regulateur: Tension_Couple/Calcule de gains ==
  data: e input; ei output; ep output
function [ei , ep]= fcn(e)

b1 = -1.1250e+03 ;
Ki=0.119;
% ei  :c'est l'erreur du couple multiplie par le gain de l'integrateur KI(du
% regulateur)
% ei  :c'est l'erreur du couple multiplie par le gain proportinnel Kp (du
% regulateur)

% le pole desire :
p = 1.5*b1;
Kp= -p/Ki ;
KI = -b1*Kp ;
ep = e*Kp ;
ei = e*KI ;

% Remarque ;
% Ki:constante du couple (couple=Ki*courant)
% KI : pour l'action integrale

== matlab function Commande_7_ReglageCascade_Hinf/RDelta_SM/Regulateur De 4 eme degree/Regulateur: Tension_Couple/Decoupleur Tension Vitess ==
  data: U4d input; U4 output; dSegma input
function U4 = fcn(U4d,dSegma)


b2 = -99.4718 ;
b3 =833.3333 ;

U4 = (U4d - b2*dSegma)/b3 ;

== matlab function Commande_7_ReglageCascade_Hinf/RDelta_SM/RD_SM2/reducteur ==
  data: alpha input; Theta output; dalpha input; dTheta output
function [Theta,dTheta]= fcn(alpha,dalpha)
%RQ : l'angle alpha est decalee de shift = -0.0651 red (problemme simmechanics)
Theta = -12*(alpha - 0.0651*[1;1;1]) ;
dTheta = -12*dalpha ;
